simulink model "Simulink_torno_est_int_obs"  (R2020a)
settings: Solver=VariableStepAuto  StartTime=0.0  StopTime=10  RelTol=1e-3
undefined symbols (not defined in the file): A_X, Ax_d, B_X, Bx_d, C_X, Cx_d, DiscIntNeverNeededParam, dt, Kix_d, Kix_I, Lx
settings Model: Creator=DELL  LastModifiedBy=DELL

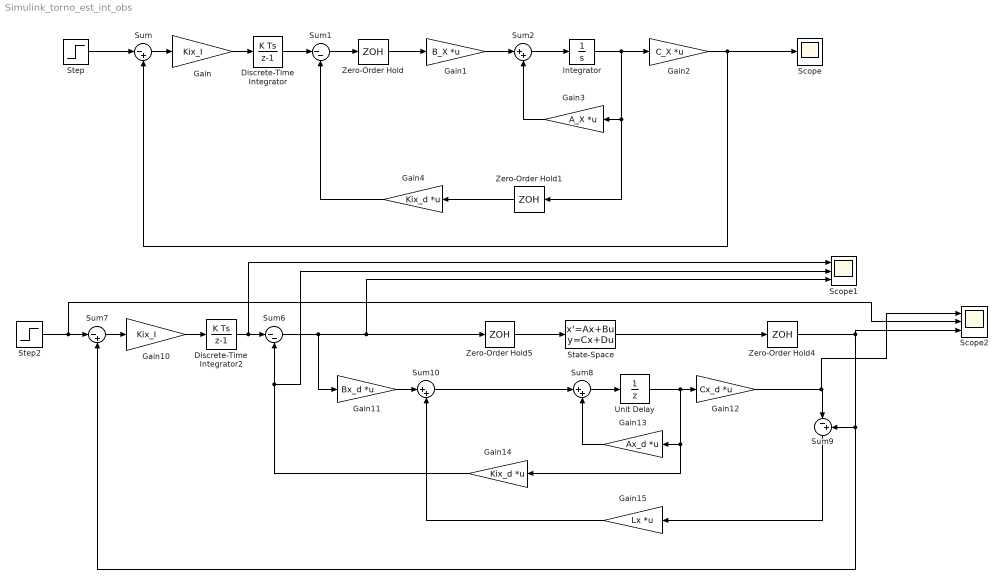
== system Simulink_torno_est_int_obs ==
  Discrete-Time Integrator : DiscreteIntegrator  SampleTime=dt  ICPrevOutput=DiscIntNeverNeededParam  ICPrevScaledInput=DiscIntNeverNeededParam
  Discrete-Time Integrator2 : DiscreteIntegrator  SampleTime=dt  ICPrevOutput=DiscIntNeverNeededParam  ICPrevScaledInput=DiscIntNeverNeededParam
  Gain : Gain  Gain=Kix_I
  Gain1 : Gain  Gain=B_X  Multiplication=Matrix(K*u)
  Gain10 : Gain  Gain=Kix_I
  Gain11 : Gain  Gain=Bx_d  Multiplication=Matrix(K*u)
  Gain12 : Gain  Gain=Cx_d  Multiplication=Matrix(K*u)
  Gain13 : Gain  Gain=Ax_d  Multiplication=Matrix(K*u)
  Gain14 : Gain  Gain=Kix_d  Multiplication=Matrix(K*u)
  Gain15 : Gain  Gain=Lx  Multiplication=Matrix(K*u)
  Gain2 : Gain  Gain=C_X  Multiplication=Matrix(K*u)
  Gain3 : Gain  Gain=A_X  Multiplication=Matrix(K*u)
  Gain4 : Gain  Gain=Kix_d  Multiplication=Matrix(K*u)
  Integrator : Integrator
  Scope : Scope
  Scope1 : Scope  NumInputPorts=3
  Scope2 : Scope  NumInputPorts=3
  State-Space : StateSpace  A=A_X  B=B_X  C=C_X  D=0  InitialCondition=0
  Step : Step  Time=2  SampleTime=dt
  Step2 : Step  Time=2  SampleTime=dt
  Sum : Sum  Inputs=|-+
  Sum1 : Sum  Inputs=|--
  Sum10 : Sum  Inputs=|++
  Sum2 : Sum  Inputs=|++
  Sum6 : Sum  Inputs=|--
  Sum7 : Sum  Inputs=|-+
  Sum8 : Sum  Inputs=|++
  Sum9 : Sum  Inputs=|-+
  Unit Delay : UnitDelay  SampleTime=-1  HasFrameUpgradeWarning=on
  Zero-Order Hold{,1,4..5} (4 alike) : ZeroOrderHold  SampleTime=dt
  wires:
  Step/1 -> Sum/1
  Sum/1 -> Gain/1
  Gain/1 -> Discrete-Time Integrator/1
  Discrete-Time Integrator/1 -> Sum1/1
  Sum1/1 -> Zero-Order Hold/1
  Zero-Order Hold/1 -> Gain1/1
  Gain1/1 -> Sum2/1
  Sum2/1 -> Integrator/1
  Integrator/1 -> Gain3/1, Zero-Order Hold1/1, Gain2/1
  Gain3/1 -> Sum2/2
  Zero-Order Hold1/1 -> Gain4/1
  Gain4/1 -> Sum1/2
  Gain2/1 -> Scope/1, Sum/2
  Sum6/1 -> Gain11/1, Scope1/3, Zero-Order Hold5/1
  Gain10/1 -> Discrete-Time Integrator2/1
  Step2/1 -> Scope2/2, Sum7/1
  Gain13/1 -> Sum8/2
  Sum10/1 -> Sum8/1
  Sum8/1 -> Unit Delay/1
  Unit Delay/1 -> Gain14/1, Gain13/1, Gain12/1
  Gain12/1 -> Scope2/1, Sum9/1
  Gain14/1 -> Scope1/2, Sum6/2
  Gain15/1 -> Sum10/2
  Gain11/1 -> Sum10/1
  Sum9/1 -> Gain15/1
  Zero-Order Hold5/1 -> State-Space/1
  Zero-Order Hold4/1 -> Sum9/2, Sum7/2, Scope2/3
  State-Space/1 -> Zero-Order Hold4/1
  Discrete-Time Integrator2/1 -> Scope1/1, Sum6/1
  Sum7/1 -> Gain10/1
